simulink model "AM_s_PWM"  (R2016a)
settings: Solver=VariableStepAuto  StartTime=0.0  StopTime=1/f_1  MaxStep=1e-5  RelTol=1e-3
InitFcn:
  | parametrizacija_as
values from neighbouring files (symbols this model uses):
  f_1 = 50    [parametrizacija_as.m]
  f_sw = f_1*15    (= 750)    [parametrizacija_as.m]
  f_vzorcenje = 50 * f_sw    (= 37500)    [parametrizacija_as.m]
  J = 0.0155    [AS_ABB.m]
  k_r = L_m/L_r    [parametrizacija_as.m]
  k_s = L_m/L_s    [parametrizacija_as.m]
  K_vu = 0.0025    [AS_ABB.m]
  L_m = 0.2342    [AS_ABB.m]
  L_r_T = L_r - L_m^2 / L_s    [parametrizacija_as.m]
  L_s_T = L_s - L_m^2 / L_r    [parametrizacija_as.m]
  M = [0 -1; 1 0]    [parametrizacija_as.m]
  p_p = 2    [AS_ABB.m]
  R_r = 2.296    [AS_ABB.m]
  R_s = 3.7    [AS_ABB.m]
  T_Z = 1/3 * [2 -1 -1; -1 2 -1; -1 -1 2]    [parametrizacija_as.m]
  V_a = V_dc / sqrt(3) * X    [Program.m]
  V_dc = 540    [parametrizacija_as.m]
  w_1 = 2*pi*f_naz    [parametrizacija_as.m]
libraries: simulink x1
settings Model: Creator=KlemenD  LastModifiedBy=matej
settings DebuggingCC: MaxConsecutiveZCsMsg=none

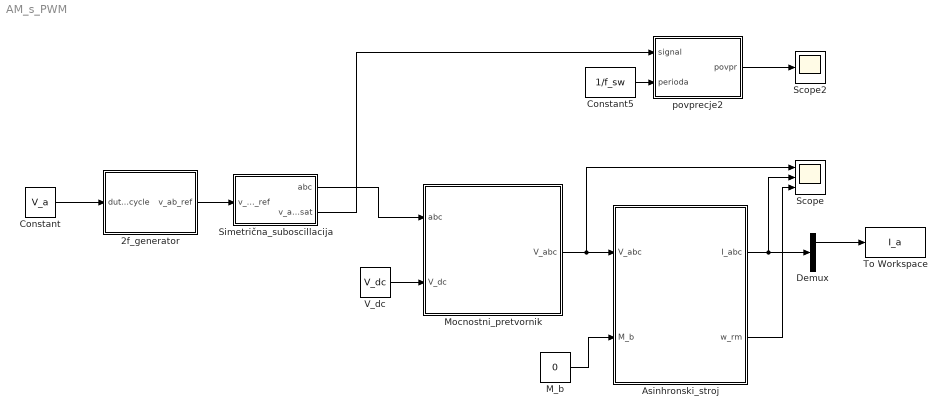
== system AM_s_PWM ==
  2f_generator : Subsystem
  Asinhronski_stroj : Subsystem
  Constant : Constant  Value=V_a
  Constant5 : Constant  Value=1/f_sw
  Demux : Demux  Outputs=3
  M_b : Constant  Value=0
  Mocnostni_pretvornik : Subsystem
  Scope : Scope  NumInputPorts=3
  Scope2 : Scope
  Simetrična_suboscillacija : Subsystem
  To Workspace : ToWorkspace  VariableName=I_a  SampleTime=1/f_vzorcenje
  V_dc : Constant  Value=V_dc
  povprecje2 : Subsystem
  wires:
  V_dc/1 -> Mocnostni_pretvornik/2(V_dc)
  Mocnostni_pretvornik/1(V_abc) -> Asinhronski_stroj/1(V_abc), Scope/1
  Asinhronski_stroj/1(I_abc) -> Demux/1, Scope/2
  M_b/1 -> Asinhronski_stroj/2(M_b)
  Asinhronski_stroj/2(w_rm) -> Scope/3
  Simetrična_suboscillacija/1(abc) -> Mocnostni_pretvornik/1(abc)
  Constant5/1 -> povprecje2/2(perioda)
  Simetrična_suboscillacija/2(v_ab_ref_sat) -> povprecje2/1(signal)
  povprecje2/1(povpr) -> Scope2/1
  2f_generator/1(v_ab_ref) -> Simetrična_suboscillacija/1(v_ab_ref)
  Constant/1 -> 2f_generator/1(duty_cycle)
  Demux/1 -> To Workspace/1

== system AM_s_PWM/2f_generator ==
  duty_cycle : Inport
  Mux2 : Mux  Inputs=2
  Product : Product  RndMeth=Zero
  Sine Wave : Sin  Frequency=2*pi*f_1  SampleTime=0
  Sine Wave1 : Sin  Frequency=2*pi*f_1  Phase=-pi/2  SampleTime=0
  v_ab_ref : Outport
  wires:
  Product/1 -> v_ab_ref/1
  Sine Wave/1 -> Mux2/1
  Sine Wave1/1 -> Mux2/2
  Mux2/1 -> Product/2
  duty_cycle/1 -> Product/1

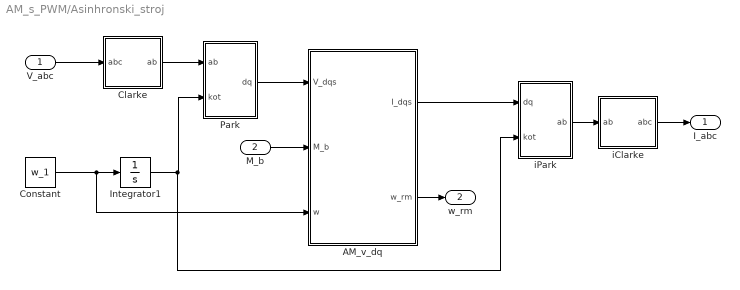
== system AM_s_PWM/Asinhronski_stroj ==
  V_abc : Inport
  M_b : Inport  Port=2
  AM_v_dq : Subsystem
  Clarke : Subsystem
  Constant : Constant  Value=w_1
  Integrator1 : Integrator
  Park : Subsystem
  iClarke : Subsystem
  iPark : Subsystem
  I_abc : Outport
  w_rm : Outport  Port=2
  wires:
  iClarke/1(abc) -> I_abc/1
  AM_v_dq/2(w_rm) -> w_rm/1
  AM_v_dq/1(I_dqs) -> iPark/1(dq)
  Park/1(dq) -> AM_v_dq/1(V_dqs)
  iPark/1(ab) -> iClarke/1(ab)
  Clarke/1(ab) -> Park/1(ab)
  V_abc/1 -> Clarke/1(abc)
  M_b/1 -> AM_v_dq/2(M_b)
  Integrator1/1 -> iPark/2(kot), Park/2(kot)
  Constant/1 -> AM_v_dq/3(w), Integrator1/1

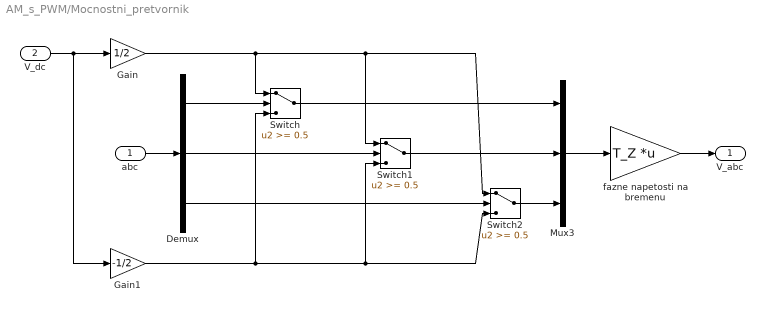
== system AM_s_PWM/Mocnostni_pretvornik ==
  abc : Inport
  V_dc : Inport  Port=2
  Demux : Demux  Outputs=3
  Gain : Gain  Gain=1/2
  Gain1 : Gain  Gain=-1/2
  Mux3 : Mux  Inputs=3
  Switch : Switch  Threshold=0.5  SaturateOnIntegerOverflow=on  InputSameDT=on
  Switch1 : Switch  Threshold=0.5  SaturateOnIntegerOverflow=on  InputSameDT=on
  Switch2 : Switch  Threshold=0.5  SaturateOnIntegerOverflow=on  InputSameDT=on
  fazne napetosti na bremenu : Gain  Gain=T_Z  Multiplication=Matrix(K*u)  SaturateOnIntegerOverflow=on  OutDataTypeStr=Inherit: Same as input  ParamDataTypeStr=Inherit: Same as input
  V_abc : Outport
  wires:
  Demux/3 -> Switch2/2
  Demux/2 -> Switch1/2
  Demux/1 -> Switch/2
  Gain1/1 -> Switch/3, Switch1/3, Switch2/3
  V_dc/1 -> Gain1/1, Gain/1
  fazne napetosti na bremenu/1 -> V_abc/1
  Mux3/1 -> fazne napetosti na bremenu/1
  Switch2/1 -> Mux3/3
  Switch1/1 -> Mux3/2
  Switch/1 -> Mux3/1
  abc/1 -> Demux/1
  Gain/1 -> Switch2/1, Switch1/1, Switch/1

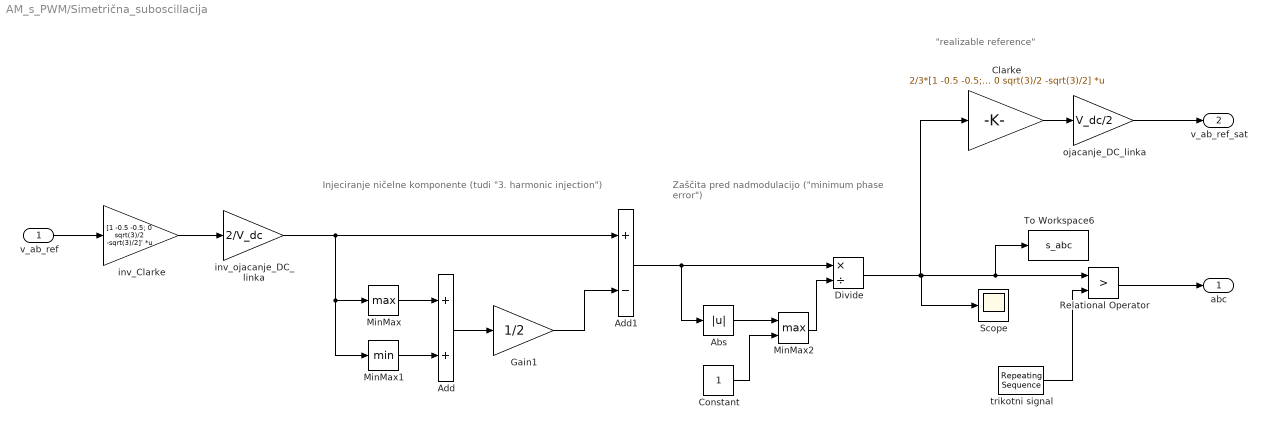
== system AM_s_PWM/Simetrična_suboscillacija ==
  note: "realizable reference"
  note: Zaščita pred nadmodulacijo
      | ("minimum phase error")
  note: Injeciranje ničelne komponente
      | (tudi "3. harmonic injection")
  v_ab_ref : Inport
  Abs : Abs
  Add : Sum
  Add1 : Sum  Inputs=+-
  Clarke : Gain  Gain=2/3*[1 -0.5 -0.5; 0 sqrt(3)/2 -sqrt(3)/2]  Multiplication=Matrix(K*u)
  Constant : Constant
  Divide : Product  Inputs=*/
  Gain1 : Gain  Gain=1/2
  MinMax : MinMax  Function=max
  MinMax1 : MinMax
  MinMax2 : MinMax  Function=max  Inputs=2
  Relational Operator : RelationalOperator  Operator=>  OutDataTypeStr=boolean  ZeroCross=off
  Scope : Scope
  To Workspace6 : ToWorkspace  VariableName=s_abc  SampleTime=1/(f_1 * 200)
  inv_Clarke : Gain  Gain=[1 -0.5 -0.5; 0 sqrt(3)/2 -sqrt(3)/2]'  Multiplication=Matrix(K*u)
  inv_ojacanje_DC_linka : Gain  Gain=2/V_dc
  ojacanje_DC_linka : Gain  Gain=V_dc/2
  trikotni signal : simulink/Sources/Repeating Sequence  rep_seq_t=[0 0.5/f_sw 1/f_sw]  rep_seq_y=[-1 1 -1]
  abc : Outport
  v_ab_ref_sat : Outport  Port=2
  wires:
  v_ab_ref/1 -> inv_Clarke/1
  inv_Clarke/1 -> inv_ojacanje_DC_linka/1
  inv_ojacanje_DC_linka/1 -> MinMax1/1, MinMax/1, Add1/1
  MinMax/1 -> Add/1
  MinMax1/1 -> Add/2
  Add/1 -> Gain1/1
  Gain1/1 -> Add1/2
  Add1/1 -> Abs/1, Divide/1
  Constant/1 -> MinMax2/2
  MinMax2/1 -> Divide/2
  Clarke/1 -> ojacanje_DC_linka/1
  ojacanje_DC_linka/1 -> v_ab_ref_sat/1
  Abs/1 -> MinMax2/1
  trikotni signal/1 -> Relational Operator/2
  Relational Operator/1 -> abc/1
  Divide/1 -> To Workspace6/1, Relational Operator/1, Scope/1, Clarke/1

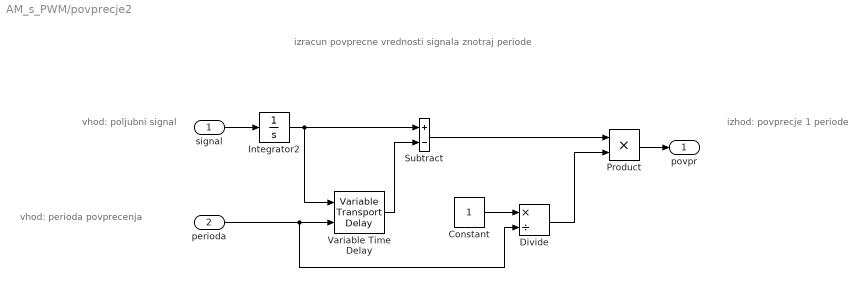
== system AM_s_PWM/povprecje2 ==
  note: izhod:
      | povprecje 1 periode
  note: vhod:
      | poljubni signal
  note: izracun povprecne vrednosti signala znotraj periode
  note: vhod:
      | perioda povprecenja
  signal : Inport
  perioda : Inport  Port=2
  Constant : Constant
  Divide : Product  Inputs=*/
  Integrator2 : Integrator
  Product : Product  RndMeth=Zero
  Subtract : Sum  Inputs=+-
  Variable Time Delay : VariableTransportDelay  MaximumDelay=10
  povpr : Outport
  wires:
  Integrator2/1 -> Subtract/1, Variable Time Delay/1
  Variable Time Delay/1 -> Subtract/2
  signal/1 -> Integrator2/1
  Product/1 -> povpr/1
  Subtract/1 -> Product/1
  perioda/1 -> Variable Time Delay/2, Divide/2
  Divide/1 -> Product/2
  Constant/1 -> Divide/1

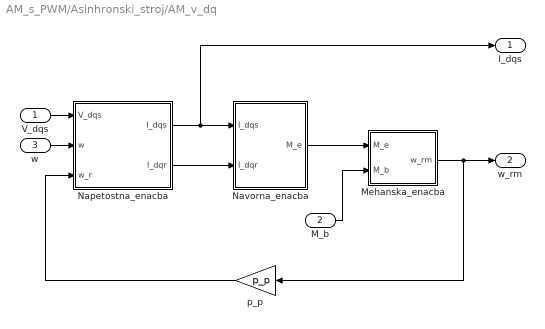
== system AM_s_PWM/Asinhronski_stroj/AM_v_dq ==
  V_dqs : Inport
  M_b : Inport  Port=2
  w : Inport  Port=3
  Mehanska_enacba : Subsystem  Description=Avtor: Mitja Nemec
  Napetostna_enacba : Subsystem
  Navorna_enacba : Subsystem
  p_p : Gain  Gain=p_p
  I_dqs : Outport
  w_rm : Outport  Port=2
  wires:
  V_dqs/1 -> Napetostna_enacba/1(V_dqs)
  Navorna_enacba/1(M_e) -> Mehanska_enacba/1(M_e)
  Napetostna_enacba/1(I_dqs) -> Navorna_enacba/1(I_dqs), I_dqs/1
  Mehanska_enacba/1(w_rm) -> p_p/1, w_rm/1
  M_b/1 -> Mehanska_enacba/2(M_b)
  p_p/1 -> Napetostna_enacba/3(w_r)
  Napetostna_enacba/2(I_dqr) -> Navorna_enacba/2(I_dqr)
  w/1 -> Napetostna_enacba/2(w)

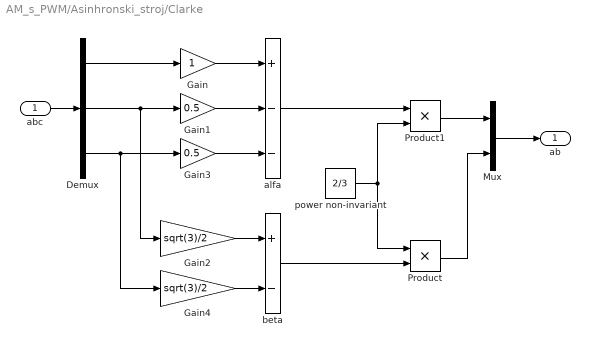
== system AM_s_PWM/Asinhronski_stroj/Clarke ==
  abc : Inport
  Demux : Demux  Outputs=3
  Gain : Gain
  Gain1 : Gain  Gain=0.5
  Gain2 : Gain  Gain=sqrt(3)/2
  Gain3 : Gain  Gain=0.5
  Gain4 : Gain  Gain=sqrt(3)/2
  Mux : Mux  Inputs=2
  Product : Product
  Product1 : Product
  alfa : Sum  Inputs=+--
  beta : Sum  Inputs=+-
  power non-invariant : Constant  Value=2/3
  ab : Outport
  wires:
  Gain/1 -> alfa/1
  Gain1/1 -> alfa/2
  Gain3/1 -> alfa/3
  Demux/1 -> Gain/1
  Demux/2 -> Gain2/1, Gain1/1
  Demux/3 -> Gain4/1, Gain3/1
  Gain2/1 -> beta/1
  Gain4/1 -> beta/2
  Product/1 -> Mux/2
  beta/1 -> Product/2
  Product1/1 -> Mux/1
  alfa/1 -> Product1/1
  power non-invariant/1 -> Product/1, Product1/2
  Mux/1 -> ab/1
  abc/1 -> Demux/1

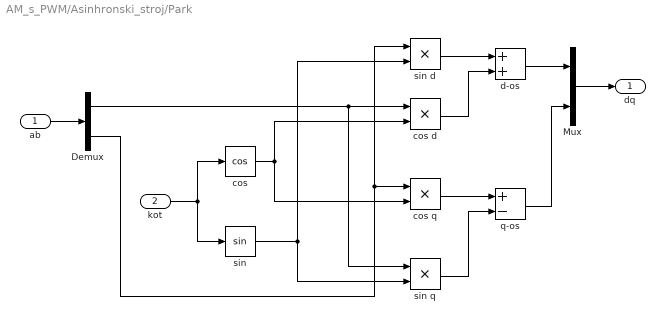
== system AM_s_PWM/Asinhronski_stroj/Park ==
  ab : Inport
  kot : Inport  Port=2
  Demux : Demux  Outputs=2
  Mux : Mux  Inputs=2
  cos : Trigonometry  Operator=cos
  cos d : Product
  cos q : Product
  d-os : Sum
  q-os : Sum  Inputs=+-
  sin : Trigonometry
  sin d : Product
  sin q : Product
  dq : Outport
  wires:
  q-os/1 -> Mux/2
  d-os/1 -> Mux/1
  Demux/2 -> sin d/1, cos q/1
  cos/1 -> cos d/2, cos q/2
  sin/1 -> sin d/2, sin q/2
  cos q/1 -> q-os/1
  sin q/1 -> q-os/2
  sin d/1 -> d-os/1
  cos d/1 -> d-os/2
  ab/1 -> Demux/1
  kot/1 -> sin/1, cos/1
  Demux/1 -> sin q/1, cos d/1
  Mux/1 -> dq/1

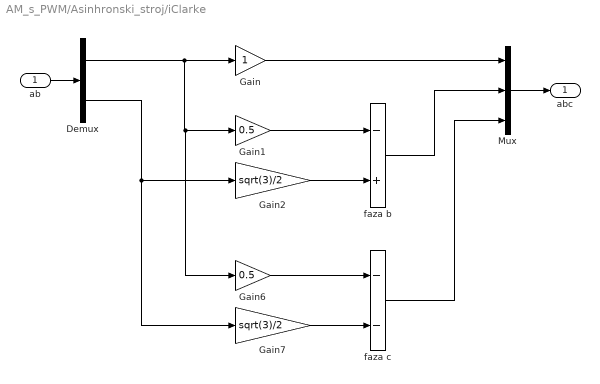
== system AM_s_PWM/Asinhronski_stroj/iClarke ==
  ab : Inport
  Demux : Demux  Outputs=2
  Gain : Gain
  Gain1 : Gain  Gain=0.5
  Gain2 : Gain  Gain=sqrt(3)/2
  Gain6 : Gain  Gain=0.5
  Gain7 : Gain  Gain=sqrt(3)/2
  Mux : Mux  Inputs=3
  faza b : Sum  Inputs=-+
  faza c : Sum  Inputs=--
  abc : Outport
  wires:
  Mux/1 -> abc/1
  ab/1 -> Demux/1
  Demux/1 -> Gain6/1, Gain1/1, Gain/1
  Gain/1 -> Mux/1
  Gain2/1 -> faza b/2
  Gain1/1 -> faza b/1
  Demux/2 -> Gain7/1, Gain2/1
  Gain7/1 -> faza c/2
  Gain6/1 -> faza c/1
  faza b/1 -> Mux/2
  faza c/1 -> Mux/3

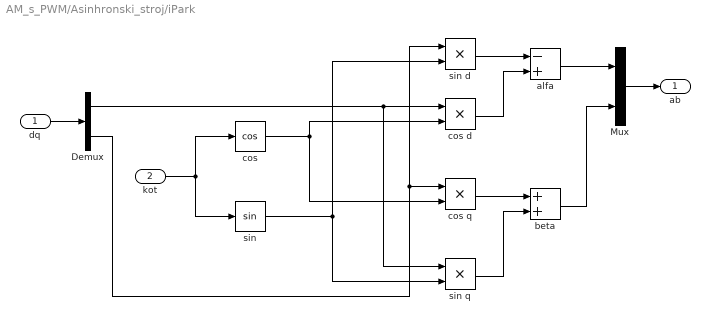
== system AM_s_PWM/Asinhronski_stroj/iPark ==
  dq : Inport
  kot : Inport  Port=2
  Demux : Demux  Outputs=2
  Mux : Mux  Inputs=2
  alfa : Sum  Inputs=-+
  beta : Sum
  cos : Trigonometry  Operator=cos
  cos d : Product
  cos q : Product
  sin : Trigonometry
  sin d : Product
  sin q : Product
  ab : Outport
  wires:
  beta/1 -> Mux/2
  alfa/1 -> Mux/1
  Demux/2 -> sin d/1, cos q/1
  cos/1 -> cos q/2, cos d/2
  sin/1 -> sin d/2, sin q/2
  cos q/1 -> beta/1
  sin q/1 -> beta/2
  sin d/1 -> alfa/1
  cos d/1 -> alfa/2
  dq/1 -> Demux/1
  kot/1 -> sin/1, cos/1
  Demux/1 -> sin q/1, cos d/1
  Mux/1 -> ab/1

== system AM_s_PWM/Asinhronski_stroj/AM_v_dq/Mehanska_enacba ==
  M_e : Inport
  M_b : Inport  Port=2
  Gain1 : Gain  Gain=1/J
  Gain3 : Gain  Gain=K_vu
  Integrator : Integrator
  Sum : Sum  Inputs=+--
  w_rm : Outport
  wires:
  Integrator/1 -> Gain3/1, w_rm/1
  M_e/1 -> Sum/1
  Sum/1 -> Gain1/1
  M_b/1 -> Sum/2
  Gain3/1 -> Sum/3
  Gain1/1 -> Integrator/1

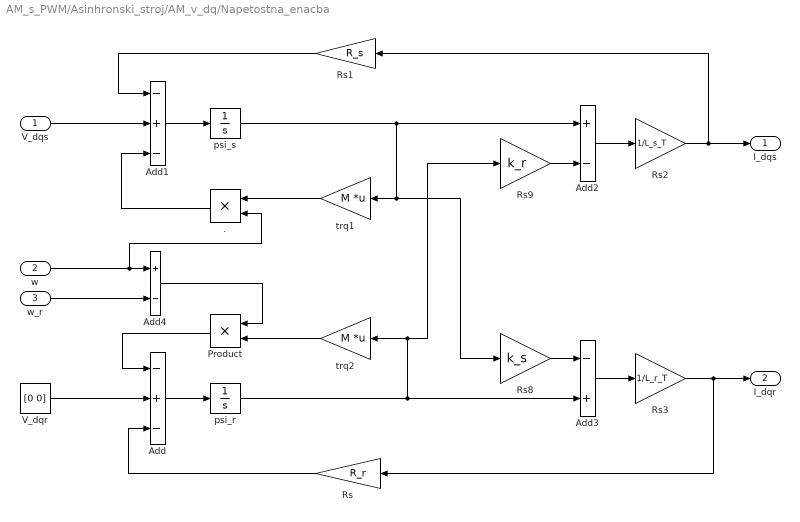
== system AM_s_PWM/Asinhronski_stroj/AM_v_dq/Napetostna_enacba ==
  V_dqs : Inport
  w : Inport  Port=2
  w_r : Inport  Port=3
  . : Product  RndMeth=Zero
  Add : Sum  Inputs=-+-
  Add1 : Sum  Inputs=-+-
  Add2 : Sum  Inputs=+-
  Add3 : Sum  Inputs=-+
  Add4 : Sum  Inputs=+-
  Product : Product  RndMeth=Zero
  Rs : Gain  Gain=R_r
  Rs1 : Gain  Gain=R_s
  Rs2 : Gain  Gain=1/L_s_T
  Rs3 : Gain  Gain=1/L_r_T
  Rs8 : Gain  Gain=k_s
  Rs9 : Gain  Gain=k_r
  V_dqr : Constant  Value=[0 0]
  psi_r : Integrator
  psi_s : Integrator
  trq1 : Gain  Gain=M  Multiplication=Matrix(K*u)
  trq2 : Gain  Gain=M  Multiplication=Matrix(K*u)
  I_dqs : Outport
  I_dqr : Outport  Port=2
  wires:
  Rs2/1 -> I_dqs/1, Rs1/1
  psi_s/1 -> Rs8/1, trq1/1, Add2/1
  ./1 -> Add1/3
  Product/1 -> Add/1
  Add/1 -> psi_r/1
  Add1/1 -> psi_s/1
  Rs1/1 -> Add1/1
  V_dqs/1 -> Add1/2
  Rs/1 -> Add/3
  V_dqr/1 -> Add/2
  psi_r/1 -> Rs9/1, trq2/1, Add3/2
  trq1/1 -> ./1
  trq2/1 -> Product/2
  w_r/1 -> Add4/2
  w/1 -> ./2, Add4/1
  Add4/1 -> Product/1
  Rs9/1 -> Add2/2
  Rs8/1 -> Add3/1
  Add2/1 -> Rs2/1
  Add3/1 -> Rs3/1
  Rs3/1 -> I_dqr/1, Rs/1

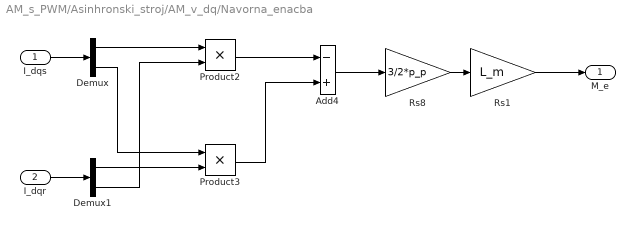
== system AM_s_PWM/Asinhronski_stroj/AM_v_dq/Navorna_enacba ==
  I_dqs : Inport
  I_dqr : Inport  Port=2
  Add4 : Sum  Inputs=-+
  Demux : Demux  Outputs=2
  Demux1 : Demux  Outputs=2
  Product2 : Product  RndMeth=Zero
  Product3 : Product  RndMeth=Zero
  Rs1 : Gain  Gain=L_m
  Rs8 : Gain  Gain=3/2*p_p
  M_e : Outport
  wires:
  Rs8/1 -> Rs1/1
  Add4/1 -> Rs8/1
  Product3/1 -> Add4/2
  Product2/1 -> Add4/1
  I_dqs/1 -> Demux/1
  I_dqr/1 -> Demux1/1
  Demux/1 -> Product2/1
  Demux1/1 -> Product3/2
  Demux/2 -> Product3/1
  Demux1/2 -> Product2/2
  Rs1/1 -> M_e/1
